simulink model "M3508_sim"  (R2017a)
settings: Solver=VariableStepAuto  StartTime=0.0  StopTime=2  RelTol=1e-3
libraries: simulink x2
settings Model: Creator=A  LastModifiedBy=A

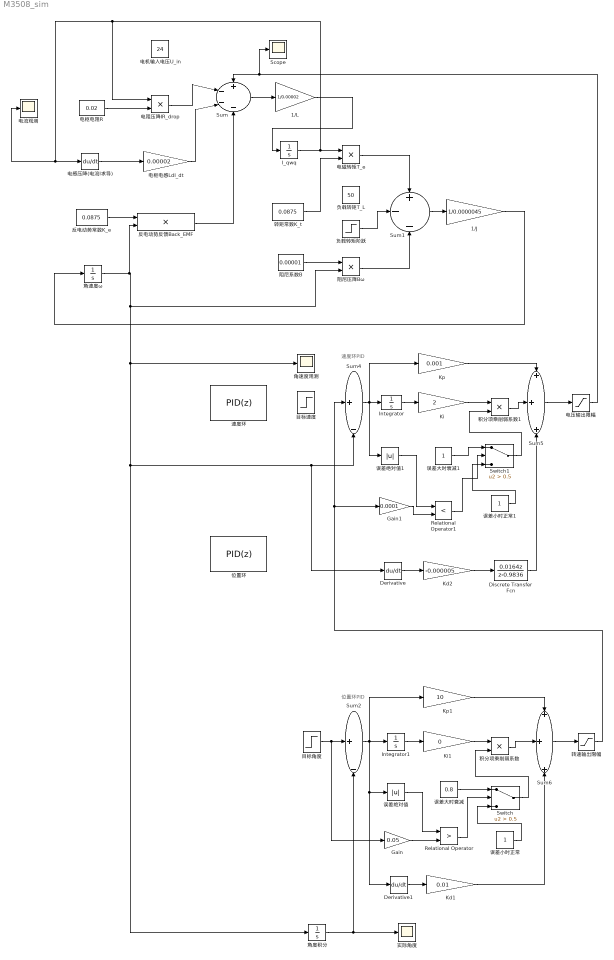
== system M3508_sim ==
  note: 速度环PID
  note: 位置环PID
  1/J : Gain  Gain=1/0.0000045
  1/L : Gain  Gain=1/0.00002
  Derivative : Derivative
  Derivative1 : Derivative
  Discrete Transfer Fcn : DiscreteTransferFcn  Numerator=[0.0164, 0]  Denominator=[1, -0.9836]  SampleTime=0.001
  Gain : Gain  Gain=0.05
  Gain1 : Gain  Gain=0.0001
  I_qwq : Integrator  ContinuousStateAttributes='position'
  Integrator : Integrator
  Integrator1 : Integrator
  Kd1 : Gain  Gain=0.01
  Kd2 : Gain  Gain=-0.000005
  Ki : Gain  Gain=2
  Ki1 : Gain  Gain=0
  Kp : Gain  Gain=0.001
  Kp1 : Gain  Gain=10
  Relational Operator : RelationalOperator  Operator=>  OutDataTypeStr=boolean  RndMeth=Simplest
  Relational Operator1 : RelationalOperator  Operator=<  OutDataTypeStr=boolean  ZeroCross=off  RndMeth=Simplest
  Scope : Scope
  Sum : Sum  Inputs=+---
  Sum1 : Sum  Inputs=+--
  Sum2 : Sum  Inputs=|+-
  Sum4 : Sum  Inputs=|+-
  Sum5 : Sum  Inputs=+++
  Sum6 : Sum  Inputs=+++
  Switch : Switch  Criteria=u2 > Threshold  Threshold=0.5
  Switch1 : Switch  Criteria=u2 > Threshold  Threshold=0.5
  位置环 : simulink/Continuous/PID Controller  Controller=PID  TimeDomain=Discrete-time  SampleTime=0.001  IntegratorMethod=Forward Euler  FilterMethod=Forward Euler  Form=Parallel  UseFilter=on  ControllerParametersSource=internal  P=5  I=2  D=0.05  N=100  InitialConditionSource=internal  InitialConditionForIntegrator=0  InitialConditionForFilter=0  ExternalReset=none  LimitOutput=on  UpperSaturationLimit=24  LowerSaturationLimit=-24  LinearizeAsGain=off  AntiWindupMode=clamping  Kb=1  TrackingMode=off  Kt=1  PParamMin=[]  PParamMax=[]  IParamMin=[]  IParamMax=[]  DParamMin=[]  DParamMax=[]  NParamMin=[]  NParamMax=[]  KbParamMin=[]  KbParamMax=[]  KtParamMin=[]  KtParamMax=[]  POutMin=[]  POutMax=[]  IOutMin=[]  IOutMax=[]  DOutMin=[]  DOutMax=[]  NOutMin=[]  NOutMax=[]  KbOutMin=[]  KbOutMax=[]  KtOutMin=[]  KtOutMax=[]  IntegratorOutMin=[]  IntegratorOutMax=[]  FilterOutMin=[]  FilterOutMax=[]  SumOutMin=[]  SumOutMax=[]  SumI1OutMin=[]  SumI1OutMax=[]  SumI2OutMin=[]  SumI2OutMax=[]  SumI3OutMin=[]  SumI3OutMax=[]  SumDOutMin=[]  SumDOutMax=[]  SaturationOutMin=[]  SaturationOutMax=[]  IntegratorContinuousStateAttributes=''  IntegratorStateMustResolveToSignalObject=off  IntegratorRTWStateStorageClass=Auto  FilterContinuousStateAttributes=''  FilterStateMustResolveToSignalObject=off  FilterRTWStateStorageClass=Auto  DifferentiatorICPrevScaledInput=0  DifferentiatorOutMin=[]  DifferentiatorOutMax=[]  InitialConditionSetting=State (most efficient)
  反电动势反馈Back_EMF : Product
  反电动势常数K_e : Constant  Value=0.0875
  实际角度 : Scope
  电压输出限幅 : Saturate  UpperLimit=24  LowerLimit=-24  ZeroCross=off
  电感压降(电流I求导) : Derivative
  电机输入电压U_in : Constant  Value=24
  电枢电感LdI_dt : Gain  Gain=0.00002
  电枢电阻R : Constant  Value=0.02
  电流观测 : Scope
  电磁转矩T_e : Product
  "电阻压降IR_drop " : Product
  目标角度 : Step  Time=0.01  After=10  SampleTime=0
  目标速度 : Step  Time=0.01  After=100  SampleTime=0
  积分项乘削弱系数 : Product
  积分项乘削弱系数1 : Product
  角度积分 : Integrator
  角速度ω : Integrator
  角速度观测 : Scope
  误差大时衰减 : Constant  Value=0.8
  误差大时衰减1 : Constant
  误差小时正常 : Constant
  误差小时正常1 : Constant
  误差绝对值 : Abs
  误差绝对值1 : Abs
  负载转矩T_L : Constant  Value=50
  负载转矩阶跃 : Step  After=5  SampleTime=0.001
  转矩常数K_t : Constant  Value=0.0875
  转速输出限幅 : Saturate  UpperLimit=250  LowerLimit=-250  ZeroCross=off
  速度环 : simulink/Continuous/PID Controller  Controller=PID  TimeDomain=Discrete-time  SampleTime=0.001  IntegratorMethod=Forward Euler  FilterMethod=Forward Euler  Form=Parallel  UseFilter=on  ControllerParametersSource=internal  P=0.06  I=5  D=0.00001  N=100  InitialConditionSource=internal  InitialConditionForIntegrator=0  InitialConditionForFilter=0  ExternalReset=none  LimitOutput=on  UpperSaturationLimit=24  LowerSaturationLimit=-24  LinearizeAsGain=off  AntiWindupMode=clamping  Kb=1  TrackingMode=off  Kt=1  PParamMin=[]  PParamMax=[]  IParamMin=[]  IParamMax=[]  DParamMin=[]  DParamMax=[]  NParamMin=[]  NParamMax=[]  KbParamMin=[]  KbParamMax=[]  KtParamMin=[]  KtParamMax=[]  POutMin=[]  POutMax=[]  IOutMin=[]  IOutMax=[]  DOutMin=[]  DOutMax=[]  NOutMin=[]  NOutMax=[]  KbOutMin=[]  KbOutMax=[]  KtOutMin=[]  KtOutMax=[]  IntegratorOutMin=[]  IntegratorOutMax=[]  FilterOutMin=[]  FilterOutMax=[]  SumOutMin=[]  SumOutMax=[]  SumI1OutMin=[]  SumI1OutMax=[]  SumI2OutMin=[]  SumI2OutMax=[]  SumI3OutMin=[]  SumI3OutMax=[]  SumDOutMin=[]  SumDOutMax=[]  SaturationOutMin=[]  SaturationOutMax=[]  IntegratorContinuousStateAttributes=''  IntegratorStateMustResolveToSignalObject=off  IntegratorRTWStateStorageClass=Auto  FilterContinuousStateAttributes=''  FilterStateMustResolveToSignalObject=off  FilterRTWStateStorageClass=Auto  DifferentiatorICPrevScaledInput=0  DifferentiatorOutMin=[]  DifferentiatorOutMax=[]  InitialConditionSetting=State (most efficient)
  阻尼压降Bω : Product
  阻尼系数B : Constant  Value=0.00001
  wires:
  反电动势常数K_e/1 -> 反电动势反馈Back_EMF/1
  电枢电阻R/1 -> "电阻压降IR_drop "/2
  电感压降(电流I求导)/1 -> 电枢电感LdI_dt/1
  "电阻压降IR_drop "/1 -> Sum/2
  电枢电感LdI_dt/1 -> Sum/3
  反电动势反馈Back_EMF/1 -> Sum/4
  Sum/1 -> 1/L/1
  转矩常数K_t/1 -> 电磁转矩T_e/2
  阻尼系数B/1 -> 阻尼压降Bω/1
  电磁转矩T_e/1 -> Sum1/1
  阻尼压降Bω/1 -> Sum1/3
  1/L/1 -> I_qwq/1
  Sum1/1 -> 1/J/1
  1/J/1 -> 角速度ω/1
  角速度ω/1 -> 角度积分/1, Derivative/1, Sum4/2, 角速度观测/1, 阻尼压降Bω/2, 反电动势反馈Back_EMF/2
  I_qwq/1 -> 电磁转矩T_e/1, 电流观测/1, 电感压降(电流I求导)/1, "电阻压降IR_drop "/1
  目标角度/1 -> Gain/1, Sum2/1
  角度积分/1 -> Sum2/2, 实际角度/1
  Derivative/1 -> Kd2/1
  Kp1/1 -> Sum6/1
  Derivative1/1 -> Kd1/1
  Ki1/1 -> 积分项乘削弱系数/1
  Integrator1/1 -> Ki1/1
  Sum2/1 -> Kp1/1, Integrator1/1, Derivative1/1, 误差绝对值/1
  Sum6/1 -> 转速输出限幅/1
  Sum5/1 -> 电压输出限幅/1
  电压输出限幅/1 -> Sum/1, Scope/1
  Kp/1 -> Sum5/1
  Ki/1 -> 积分项乘削弱系数1/1
  误差绝对值/1 -> Relational Operator/1
  Gain/1 -> Relational Operator/2
  误差大时衰减/1 -> Switch/1
  误差小时正常/1 -> Switch/3
  Relational Operator/1 -> Switch/2
  Switch/1 -> 积分项乘削弱系数/2
  积分项乘削弱系数/1 -> Sum6/2
  Switch1/1 -> 积分项乘削弱系数1/2
  Sum4/1 -> Integrator/1, Kp/1, 误差绝对值1/1
  误差小时正常1/1 -> Switch1/3
  Relational Operator1/1 -> Switch1/2
  Gain1/1 -> Relational Operator1/2
  误差大时衰减1/1 -> Switch1/1
  误差绝对值1/1 -> Relational Operator1/1
  积分项乘削弱系数1/1 -> Sum5/2
  Integrator/1 -> Ki/1
  Kd2/1 -> Discrete Transfer Fcn/1
  Discrete Transfer Fcn/1 -> Sum5/3
  转速输出限幅/1 -> Gain1/1, Sum4/1
  Kd1/1 -> Sum6/3
  负载转矩阶跃/1 -> Sum1/2
